simulink library "DesignTemplateLib"  (R2022a)
settings: Solver=VariableStepAuto  StartTime=0.0  StopTime=10.0  RelTol=1e-3
settings Model: Creator=sawad  LastModifiedBy=sawad
settings DebuggingCC: UnconnectedInputMsg=warning  UnconnectedOutputMsg=warning  UnconnectedLineMsg=warning
settings RTWCC: DLArmComputeVersion=19.05

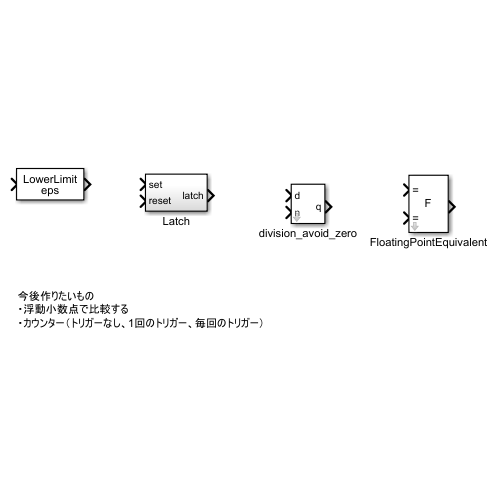
[thumbnail: Simulink's stored preview of the top-level diagram]
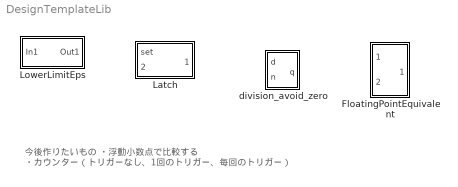
== system DesignTemplateLib ==
  note: 今後作りたいもの
      | ・浮動小数点で比較する
      | ・カウンター（トリガーなし、1回のトリガー、毎回のトリガー）
  FloatingPointEquivalent : Subsystem  mask(浮動小数点の等価判定){Value=eps}
      mask prompts: Value "許容範囲(tolerance level)"
      mask help: 第1入力と第2入力が許容誤差以内で等しい場合、等価と判定し、Trueを出力します。
      mask TypeOptions Value: Constant/Value
      mask DialogControl ParameterGroupVar Prompt: パラメーター
      mask Display:
      | port_label('input', 1,'=');
      | port_label('input', 2,'=');
      | disp('F');
  Latch : Subsystem
  LowerLimitEps : Subsystem
      mask Display: disp('LowerLimit\neps')
  division_avoid_zero : Subsystem  mask(除算（ゼロ割対策済）){MINIMUM_ERR=255, MAX_VALUE=1e-7}
      mask prompts: MINIMUM_ERR "除数が最小誤差未満時の出力値"; MAX_VALUE "最小誤差"
      mask help: 除数が最小誤差未満の場合、設定された値を出力します。
      mask DialogControl ParameterGroupVar Prompt: パラメーター

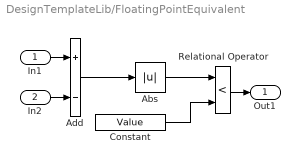
== system DesignTemplateLib/FloatingPointEquivalent ==
  In1 : Inport
  In2 : Inport  Port=2
  Abs : Abs  SaturateOnIntegerOverflow=off
  Add : Sum  Inputs=+-
  Constant : Constant  Description=説明を加えてください  Value=Value
  Relational Operator : RelationalOperator  Operator=<  OutDataTypeStr=boolean  RndMeth=Simplest  InputSameDT=off
  Out1 : Outport
  wires:
  Constant/1 -> Relational Operator/2
  Relational Operator/1 -> Out1/1
  Abs/1 -> Relational Operator/1
  In1/1 -> Add/1
  Add/1 -> Abs/1
  In2/1 -> Add/2

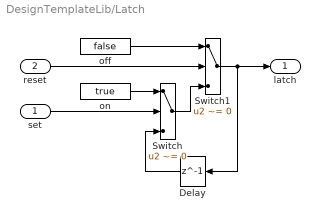
== system DesignTemplateLib/Latch ==
  set : Inport
  reset : Inport  Port=2
  Delay : Delay  DelayLength=1  InitialCondition=false
      settings: AttributesFormatString=InitialCondition=%<InitialCondition>
  Switch : Switch  Criteria=u2 ~= 0  SaturateOnIntegerOverflow=off  InputSameDT=off
  Switch1 : Switch  Criteria=u2 ~= 0  SaturateOnIntegerOverflow=off  InputSameDT=off
  off : Constant  Value=false
  on : Constant  Value=true
  latch : Outport
  wires:
  Switch/1 -> Switch1/3
  Switch1/1 -> latch/1, Delay/1
  Delay/1 -> Switch/3
  set/1 -> Switch/2
  reset/1 -> Switch1/2
  off/1 -> Switch1/1
  on/1 -> Switch/1

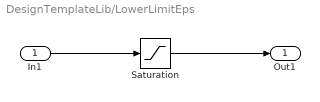
== system DesignTemplateLib/LowerLimitEps ==
  In1 : Inport
  Saturation : Saturate  UpperLimit=inf  LowerLimit=eps
      settings: AttributesFormatString=|
      | UpperLimit=%<UpperLimit>
      | LowerLimit=%<LowerLimit>
  Out1 : Outport
  wires:
  In1/1 -> Saturation/1
  Saturation/1 -> Out1/1

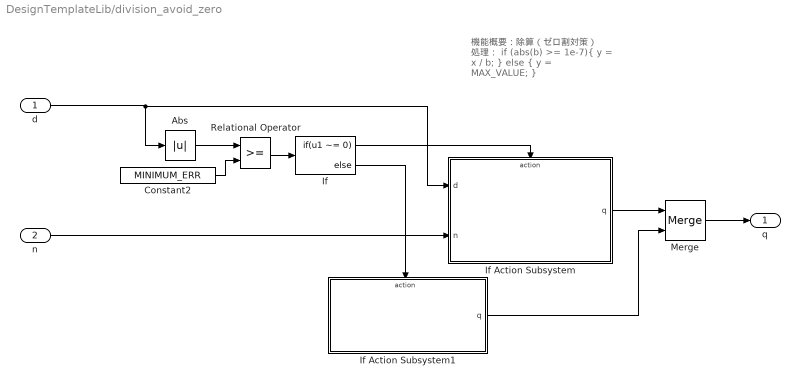
== system DesignTemplateLib/division_avoid_zero ==
  note: 機能概要：除算（ゼロ割対策）
      | 処理：
      | if (abs(b) >= 1e-7){
      | y = x / b;
      | } else {
      | y = MAX_VALUE;
      | }
  d : Inport
  n : Inport  Port=2
  Abs : Abs  SaturateOnIntegerOverflow=off
  Constant2 : Constant  Value=MINIMUM_ERR
  If : If  IfExpression=u1 ~= 0
  If Action Subsystem : Subsystem  TreatAsAtomicUnit=on
  If Action Subsystem1 : Subsystem  TreatAsAtomicUnit=on
  Merge : Merge
  Relational Operator : RelationalOperator  OutDataTypeStr=boolean  RndMeth=Simplest  InputSameDT=off
  q : Outport
  wires:
  Merge/1 -> q/1
  d/1 -> If Action Subsystem/1(d), Abs/1
  If/1 -> If Action Subsystem/Action
  If Action Subsystem1/1(q) -> Merge/2
  If/2 -> If Action Subsystem1/Action
  Constant2/1 -> Relational Operator/2
  If Action Subsystem/1(q) -> Merge/1
  Relational Operator/1 -> If/1
  n/1 -> If Action Subsystem/2(n)
  Abs/1 -> Relational Operator/1

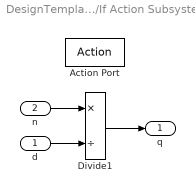
== system DesignTemplateLib/division_avoid_zero/If Action Subsystem ==
  d : Inport
  n : Inport  Port=2
  Action Port : ActionPort
  Divide1 : Product  Inputs=*/
  q : Outport
  wires:
  d/1 -> Divide1/2
  Divide1/1 -> q/1
  n/1 -> Divide1/1

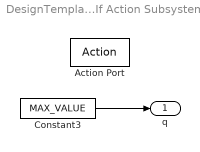
== system DesignTemplateLib/division_avoid_zero/If Action Subsystem1 ==
  Action Port : ActionPort
  Constant3 : Constant  Value=MAX_VALUE
  q : Outport
  wires:
  Constant3/1 -> q/1
